simulink model "lab1_2"  (R2016a)
settings: Solver=VariableStepAuto  StartTime=0.0  StopTime=25  RelTol=1e-3
settings Model: Creator=ms36124  LastModifiedBy=ms36124

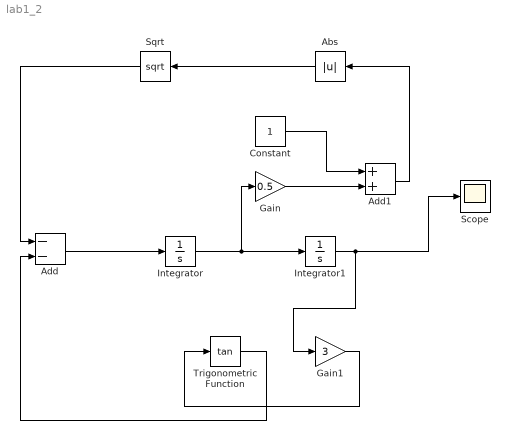
== system lab1_2 ==
  Abs : Abs
  Add : Sum  Inputs=--
  Add1 : Sum
  Constant : Constant
  Gain : Gain  Gain=0.5
  Gain1 : Gain  Gain=3
  Integrator : Integrator
  Integrator1 : Integrator  InitialCondition=1
  Scope : Scope
  Sqrt : Sqrt  SaturateOnIntegerOverflow=on
  Trigonometric Function : Trigonometry  Operator=tan
  wires:
  Add/1 -> Integrator/1
  Integrator/1 -> Gain/1, Integrator1/1
  Gain/1 -> Add1/2
  Constant/1 -> Add1/1
  Integrator1/1 -> Scope/1, Gain1/1
  Gain1/1 -> Trigonometric Function/1
  Trigonometric Function/1 -> Add/2
  Add1/1 -> Abs/1
  Abs/1 -> Sqrt/1
  Sqrt/1 -> Add/1
